simulink model "Sim_Knickarmroboter_Backup1_AndreasPaul"  (R2024a)
settings: Solver=VariableStepAuto  StartTime=0.0  StopTime=10.0  RelTol=1e-3
values from neighbouring files (symbols this model uses):
  F_s1 = 1    [Reibmoment02_TESTFILE.m]
  mu_v1 = 0.1    [Reibmoment02_TESTFILE.m]
undefined symbols (not defined in the file or in its folder): F_s2, g, I1, I2, l1, l2, m1, m2, mu_v2
libraries: slpidlib x1
settings Model: Creator=apaul  LastModifiedBy=apaul

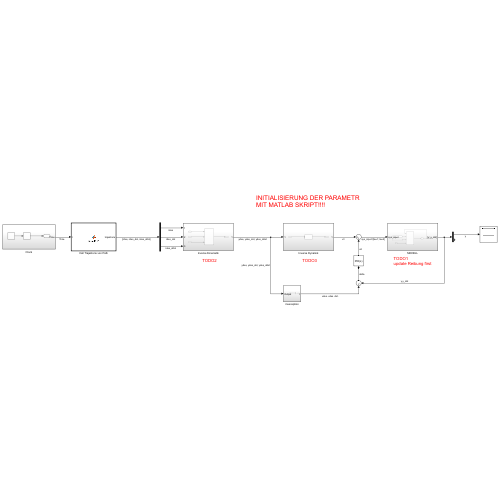
[thumbnail: Simulink's stored preview of the top-level diagram]
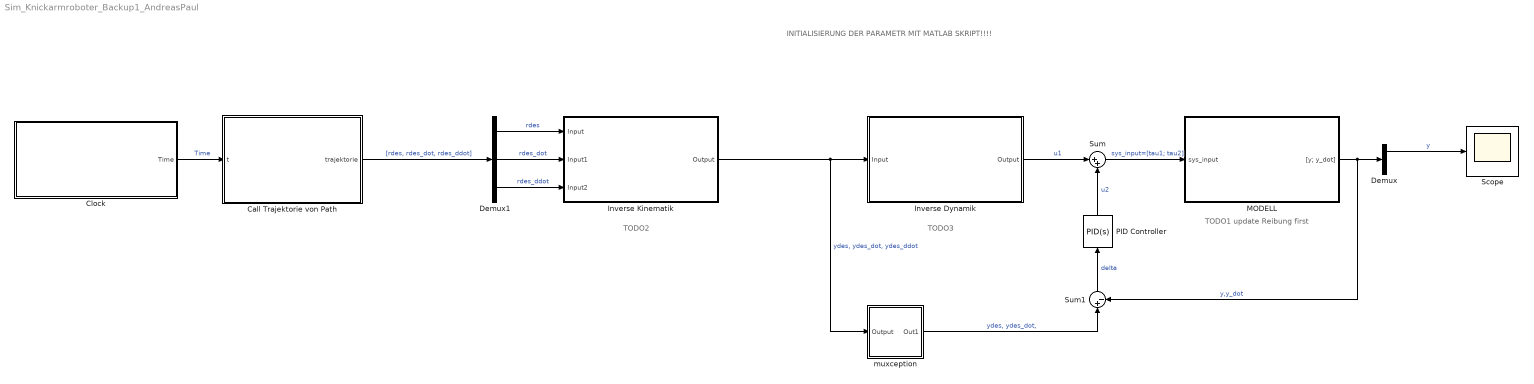
== system Sim_Knickarmroboter_Backup1_AndreasPaul ==
  note: TODO2
  note: INITIALISIERUNG DER PARAMETR MIT MATLAB SKRIPT!!!!
  note: TODO3
  note: TODO1
      | update Reibung first
  Call Trajektorie von Path : MATLAB Function  TreatAsAtomicUnit=on
  Clock : Subsystem
  Demux : Demux  Outputs=2
  Demux1 : Demux  Outputs=3
  Inverse Dynamik : Subsystem
  Inverse Kinematik : Subsystem
  MODELL : Subsystem
  PID Controller : slpidlib/PID Controller  Controller=PID  Form=Parallel  TimeDomain=Continuous-time  UseExternalTs=off  SampleTime=-1  IntegratorMethod=Forward Euler  FilterMethod=Forward Euler  ControllerParametersSource=internal  P=1  I=1  UseKiTs=off  D=0  UseExternalDerivativeSource=off  N=100  UseFilter=on  TunerSelectOption=Transfer Function Based (PID Tuner App)  InitialConditionSource=internal  InitialConditionForIntegrator=0  InitialConditionForFilter=0  DifferentiatorICPrevScaledInput=0  ExternalReset=none  TrackingMode=off  Kt=1  LimitOutput=off  SatLimitsSource=internal  UpperSaturationLimit=inf  LowerSaturationLimit=-inf  LinearizeAsGain=on  AntiWindupMode=none  Kb=1  LimitIntegrator=off  UpperIntegratorSaturationLimit=inf  LowerIntegratorSaturationLimit=-inf  POutMin=[]  POutMax=[]  IOutMin=[]  IOutMax=[]  DOutMin=[]  DOutMax=[]  NOutMin=[]  NOutMax=[]  SumOutMin=[]  SumOutMax=[]  SaturationOutMin=[]  SaturationOutMax=[]  PParamMin=[]  PParamMax=[]  IParamMin=[]  IParamMax=[]  DParamMin=[]  DParamMax=[]  NParamMin=[]  NParamMax=[]  KbParamMin=[]  KbParamMax=[]  KtParamMin=[]  KtParamMax=[]  KbOutMin=[]  KbOutMax=[]  KtOutMin=[]  KtOutMax=[]  IntegratorOutMin=[]  IntegratorOutMax=[]  FilterOutMin=[]  FilterOutMax=[]  SumI1OutMin=[]  SumI1OutMax=[]  SumI2OutMin=[]  SumI2OutMax=[]  SumI3OutMin=[]  SumI3OutMax=[]  SumI4OutMin=[]  SumI4OutMax=[]  SumDOutMin=[]  SumDOutMax=[]  DifferentiatorOutMin=[]  DifferentiatorOutMax=[]  FilterDiffOutCoefMin=[]  FilterDiffOutCoefMax=[]  ReciprocalOutMin=[]  ReciprocalOutMax=[]  SumDenOutMin=[]  SumDenOutMax=[]  SumNumOutMin=[]  SumNumOutMax=[]  DivideOutMin=[]  DivideOutMax=[]  UdiffTsProdOutMin=[]  UdiffTsProdOutMax=[]  NTsProdOutMin=[]  NTsProdOutMax=[]  UintegralTsProdOutMin=[]  UintegralTsProdOutMax=[]  UngainTsProdOutMin=[]  UngainTsProdOutMax=[]  ClampingZeroOutDataTypeStr=Inherit: Inherit via back propagation  ClampingZeroOutMin=[]  ClampingZeroOutMax=[]  FilterDenConstantOutDataTypeStr=Inherit: Inherit via back propagation  FilterDenConstantOutMin=[]  FilterDenConstantOutMax=[]  PCopyOutDataTypeStr=Inherit: Inherit via back propagation  PCopyOutMin=[]  PCopyOutMax=[]  NCopyOutDataTypeStr=Inherit: Inherit via back propagation  NCopyOutMin=[]  NCopyOutMax=[]  IntegratorContinuousStateAttributes=''  IntegratorStateMustResolveToSignalObject=off  IntegratorRTWStateStorageClass=Auto  FilterContinuousStateAttributes=''  FilterStateMustResolveToSignalObject=off  FilterRTWStateStorageClass=Auto  ParallelPVariant=InternalParameters  IdealPVariant=Disabled  IVariant=InternalParameters  DVariant=InternalParameters  IntegratorVariant=Continuous  SatVariant=Disabled  AWVariant=Passthrough  PCopyVariant=Disabled  TRVariant=Disabled  FdbkBlocksVariant=Forward  IdealPFdbkVariant=Disabled  SatFdbkVariant=Disabled  DerivativeFilterVariant=ContFilter  NVariant=InternalParameters  NCopyVariant=Disabled  FilterICVariant=InternalICsFilter  IntegratorICVariant=InternalICs  ExternalResetVariant=Disabled  TRSumVariant=Passthrough  SumFdbkVariant=Disabled  SumVariant=Sum_PID  TsampFilterVariant=InternalTs  TsampNgainVariant=Passthrough  TsampIntegralVariant=Disabled_SignalSpec  ExternalSaturationOutDataTypeStr=Inherit: Same as second input  DerivativeSourceVariant=ErrorSignal
  Scope : Scope
  Sum : Sum  Inputs=|++
  Sum1 : Sum  Inputs=|+-
  muxception : Subsystem
  wires:
  Sum/1 -> MODELL/1(sys_input)  "sys_input=[tau1; tau2]"
  PID Controller/1 -> Sum/2  "u2"
  Sum1/1 -> PID Controller/1  "delta"
  MODELL/1("[y; y_dot]") -> Demux/1, Sum1/2  "y,y_dot"
  Inverse Kinematik/1(Output) -> Inverse Dynamik/1(Input), muxception/1(Output)  "ydes, ydes_dot, ydes_ddot"
  Inverse Dynamik/1(Output) -> Sum/1  "u1"
  Demux/1 -> Scope/1  "y"
  muxception/1(Out1) -> Sum1/1  "ydes, ydes_dot,"
  Call Trajektorie von Path/1(trajektorie) -> Demux1/1  "[rdes, rdes_dot, rdes_ddot]"
  Demux1/3 -> Inverse Kinematik/3(Input2)  "rdes_ddot"
  Demux1/2 -> Inverse Kinematik/2(Input1)  "rdes_dot"
  Demux1/1 -> Inverse Kinematik/1(Input)  "rdes"
  Clock/1(Time) -> Call Trajektorie von Path/1(t)  "Time"

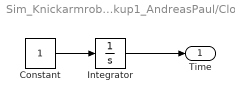
== system Sim_Knickarmroboter_Backup1_AndreasPaul/Clock ==
  Constant : Constant
  Integrator : Integrator
  Time : Outport
  wires:
  Constant/1 -> Integrator/1
  Integrator/1 -> Time/1

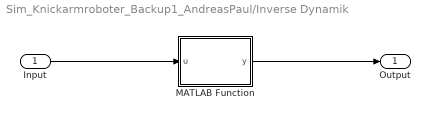
== system Sim_Knickarmroboter_Backup1_AndreasPaul/Inverse Dynamik ==
  Input : Inport
  MATLAB Function : MATLAB Function  TreatAsAtomicUnit=on
  Output : Outport
  wires:
  Input/1 -> MATLAB Function/1(u)
  MATLAB Function/1(y) -> Output/1

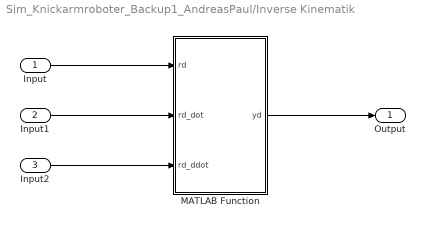
== system Sim_Knickarmroboter_Backup1_AndreasPaul/Inverse Kinematik ==
  Input : Inport
  Input1 : Inport  Port=2
  Input2 : Inport  Port=3
  MATLAB Function : MATLAB Function  TreatAsAtomicUnit=on
  Output : Outport
  wires:
  Input/1 -> MATLAB Function/1(rd)
  MATLAB Function/1(yd) -> Output/1
  Input1/1 -> MATLAB Function/2(rd_dot)
  Input2/1 -> MATLAB Function/3(rd_ddot)

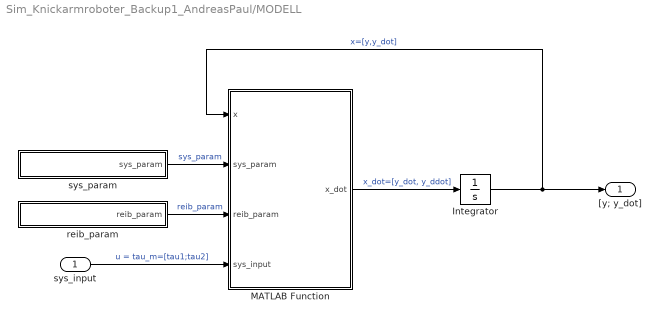
== system Sim_Knickarmroboter_Backup1_AndreasPaul/MODELL ==
  sys_input : Inport
  Integrator : Integrator
  MATLAB Function : MATLAB Function  TreatAsAtomicUnit=on
  reib_param : Subsystem
  sys_param : Subsystem
  "[y; y_dot]" : Outport
  wires:
  MATLAB Function/1(x_dot) -> Integrator/1  "x_dot=[y_dot, y_ddot]"
  Integrator/1 -> MATLAB Function/1(x), "[y; y_dot]"/1  "x=[y,y_dot]"
  sys_input/1 -> MATLAB Function/4(sys_input)  "u = tau_m=[tau1;tau2]"
  sys_param/1(sys_param) -> MATLAB Function/2(sys_param)  "sys_param"
  reib_param/1(reib_param) -> MATLAB Function/3(reib_param)  "reib_param"

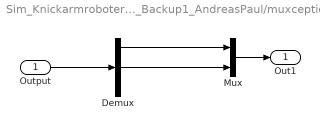
== system Sim_Knickarmroboter_Backup1_AndreasPaul/muxception ==
  Output : Inport
  Demux : Demux  Outputs=3
  Mux : Mux  Inputs=2
  Out1 : Outport
  wires:
  Output/1 -> Demux/1
  Demux/1 -> Mux/1
  Demux/2 -> Mux/2
  Mux/1 -> Out1/1

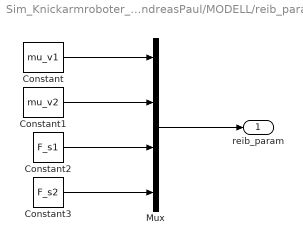
== system Sim_Knickarmroboter_Backup1_AndreasPaul/MODELL/reib_param ==
  Constant : Constant  Value=mu_v1
  Constant1 : Constant  Value=mu_v2
  Constant2 : Constant  Value=F_s1
  Constant3 : Constant  Value=F_s2
  Mux : Mux
  reib_param : Outport
  wires:
  Constant3/1 -> Mux/4
  Constant2/1 -> Mux/3
  Constant1/1 -> Mux/2
  Constant/1 -> Mux/1
  Mux/1 -> reib_param/1

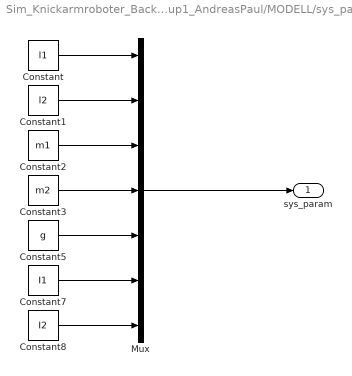
== system Sim_Knickarmroboter_Backup1_AndreasPaul/MODELL/sys_param ==
  Constant : Constant  Value=l1
  Constant1 : Constant  Value=l2
  Constant2 : Constant  Value=m1
  Constant3 : Constant  Value=m2
  Constant5 : Constant  Value=g
  Constant7 : Constant  Value=I1
  Constant8 : Constant  Value=I2
  Mux : Mux  Inputs=7
  sys_param : Outport
  wires:
  Constant8/1 -> Mux/7
  Constant7/1 -> Mux/6
  Constant3/1 -> Mux/4
  Constant2/1 -> Mux/3
  Constant1/1 -> Mux/2
  Constant/1 -> Mux/1
  Mux/1 -> sys_param/1
  Constant5/1 -> Mux/5

== matlab function Sim_Knickarmroboter_Backup1_AndreasPaul/Inverse Dynamik/MATLAB Function ==
  data: u input; y output
function y = fcn(u)

y = u;

== matlab function Sim_Knickarmroboter_Backup1_AndreasPaul/MODELL/MATLAB Function ==
  data: x input; sys_param input; reib_param input; x_dot output; sys_input input
function x_dot = fcn(x, sys_param, reib_param, sys_input)
%x(1:3)=y
%x(4:6)=y_dot
M = MassMatrix(x(1:3), sys_param, sys_input);
D = DMatrix(x(1:3), x(4:6), sys_param, sys_input, reib_param);
G = GVector(x(1:3), sys_param, sys_input, reib_param);
tau_R = CALCtau_R(x(1:3), x(4:6), sys_param, sys_input, reib_param);

%State Space System
x_dot = 123;
end

== matlab function Sim_Knickarmroboter_Backup1_AndreasPaul/Inverse Kinematik/MATLAB Function ==
  data: rd input; yd output; rd_dot input; rd_ddot input
function yd = fcn(rd,rd_dot,rd_ddot)

%Initialisierung
syms alpha beta alpha_dot beta_dot alpha_ddot beta_ddot
y = [alpha; beta];
y_dot = [alpha_dot; beta_dot];
y_ddot = [alpha_ddot; beta_ddot];
T_0EF = T_0EF_fcn(alpha, beta, l1, l2);


r = T_0EF(1:3,4);


%Ort
eq1 = r == rd;

q = solve(eq1, alpha, beta);
alpha_sol = double(q.alpha(1));
beta_sol = double(q.beta(1));
y_new = [alpha_sol; beta_sol];

%Geschwindigkeit
%Notiz: r ist in inertial coordiantes? KA deutsch lol, deswegen physical
%derr. gleich numerischer derr. 
%und nutze Kettenregel: r_dot = (dr/dy)*y_dot
J = jacobian(r,y);
r_dot = J * y_dot;
r_dot = subs(r_dot, y, y_new);

eq2 = r_dot == rd_dot;

q_dot = solve(eq2, alpha_dot, beta_dot);
alpha_dot_sol = double(q_dot.alpha_dot(1));
beta_dot_sol = double(q_dot.beta_dot(1));
y_dot_new = [alpha_dot_sol; beta_dot_sol];

%Beschleunigung
%erneut Kettenregel:
%r_ddot = J_dot*y_dot + J*y_ddot
%Da J eine Matrix ist, kann man nicht einfach mit jacobian Befehl arbeiten,
%muss Elementweise erledigt werden.
J_dot = sym(zeros(size(J))); 
for i = 1:size(J, 1)
    for j = 1:size(J, 2)
        J_dot(i, j) = jacobian(J(i, j), y) * y_dot;
    end
end

r_ddot = J_dot * y_dot + J * y_ddot;
r_ddot = subs(r_ddot, [y;y_dot], [y_new; y_dot_new]);

eq3 = r_ddot == rd_ddot;

q_ddot = solve(eq3, alpha_ddot, beta_ddot);
alpha_ddot_sol = double(q_ddot.alpha_ddot(1));
beta_ddot_sol = double(q_ddot.beta_ddot(1));
y_ddot_new = [alpha_ddot_sol; beta_ddot_sol];

yd = [y_new; y_dot_new; y_ddot_new];
end

== matlab function Sim_Knickarmroboter_Backup1_AndreasPaul/Call Trajektorie von Path ==
  data: trajektorie output; t input
function trajektorie = trajektorie(t)
%Trajektorie
%    TRAJEKTORIE = Trajektorie(T)

%    This function was generated by the Symbolic Math Toolbox version 24.1.
%    07-Jan-2025 10:14:32

t2 = t.^2;
t3 = t.^3;
t4 = t.*7.030674334031603e-2;
t5 = t.*5.130385555576637e-2;
t6 = t2.*2.565192777788319e-2;
t7 = t2.*3.515337167015802e-2;
trajektorie = [t3.*1.171779055671934e-2-t7;t3.*8.550642592627729e-3-t6-5.7e+1./2.5e+2;0.0;-t4+t7;-t5+t6;0.0;t4-7.030674334031603e-2;t5-5.130385555576637e-2;0.0];
end
